simulink model "gridforMV"  (R2015b)
settings: Solver=FixedStepDiscrete  StartTime=0.0  StopTime=10.0  RelTol=1e-3
PreLoadFcn:
  | Ts=50e-6;
InitFcn:
  | Ts=50e-6;
undefined symbols (not defined in the file or in its folder): D1, Delta, DiscIntNeverNeededParam
libraries: powerlib x19, powerlib_meascontrol x5
Description:
  | Copyright 2008-2015 The MathWorks, Inc.
settings Model: FPTRunName=Active  Creator=MathWorks  LastModifiedBy=Eren
settings DataIOCC: SaveFormat=Array  SignalLoggingSaveFormat=ModelDataLogs
settings OptimizationCC: ExpressionDepthLimit=2147483647
settings DebuggingCC: UnderspecifiedInitializationDetection=Classic  MergeDetectMultiDrivingBlocksExec=none  SolverPrmCheckMsg=warning  FcnCallInpInsideContextMsg=EnableAllAsWarning  StateNameClashWarn=warning
settings HardwareCC: ProdBitPerPointer=32  ProdLargestAtomicFloat=None  ProdIntDivRoundTo=Undefined  ProdEndianess=Unspecified  ProdWordSize=32  ProdHWDeviceType=32-bit Generic
settings GRTTargetCC: GeneratePreprocessorConditionals=Disable all  CombineOutputUpdateFcns=off  GRTInterface=on
settings ConfigComp: CovModelRefEnable=Off  CovSFcnEnable=off

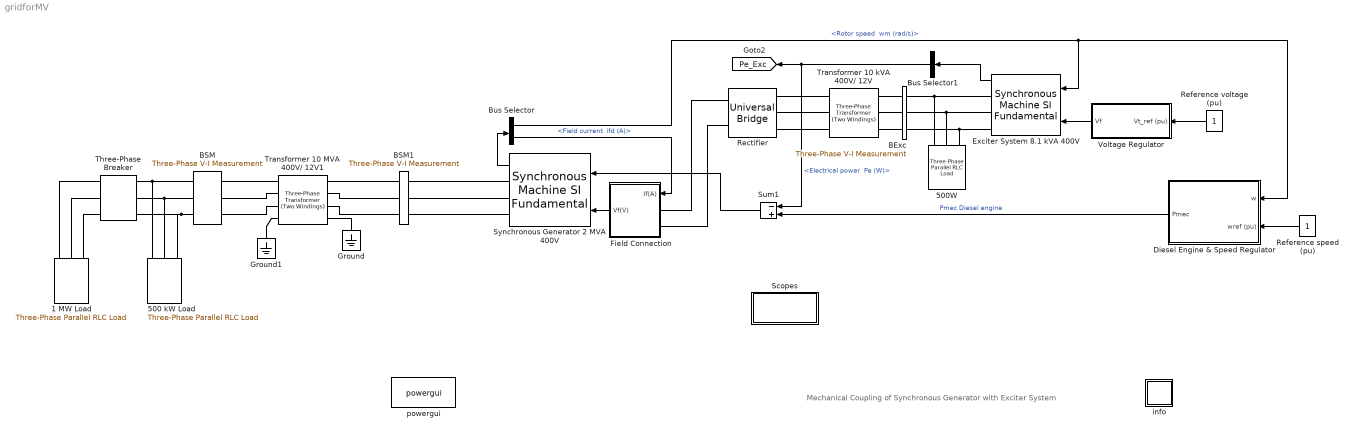
== system gridforMV ==
  note: Mechanical Coupling of Synchronous Generator with Exciter System
  "1 MW Load " : powerlib/Elements/Three-Phase Parallel RLC Load  LConnTagsString=A|B|C  Configuration=Y (grounded)  NominalVoltage=10800*sqrt(3)  Vabc=[1e3 1e3 1e3]  Vabcp=[1e3 1e3 1e3]  NominalFrequency=50  UnbalancedPower=off  ActivePower=1e6  InductivePower=0  CapacitivePower=0  Pabc=[10e3 9e3 11e3]  QLabc=[100 90 110]  QCabc=[100 90 110]  Pabcp=[10e3 9e3 11e3]  QLabcp=[100 90 110]  QCabcp=[100 90 110]  Measurements=None  LoadType=constant Z
  500 kW Load : powerlib/Elements/Three-Phase Parallel RLC Load  LConnTagsString=A|B|C  Configuration=Y (grounded)  NominalVoltage=10800*sqrt(3)  Vabc=[1e3 1e3 1e3]  Vabcp=[1e3 1e3 1e3]  NominalFrequency=50  UnbalancedPower=off  ActivePower=500e3  InductivePower=0  CapacitivePower=0  Pabc=[10e3 9e3 11e3]  QLabc=[100 90 110]  QCabc=[100 90 110]  Pabcp=[10e3 9e3 11e3]  QLabcp=[100 90 110]  QCabcp=[100 90 110]  Measurements=None  LoadType=constant Z
  500W : powerlib/Elements/Three-Phase Parallel RLC Load  LConnTagsString=A|B|C  Configuration=Y (grounded)  NominalVoltage=400  Vabc=[1e3 1e3 1e3]  Vabcp=[1e3 1e3 1e3]  NominalFrequency=50  UnbalancedPower=off  ActivePower=500  InductivePower=0  CapacitivePower=0  Pabc=[10e3 9e3 11e3]  QLabc=[100 90 110]  QCabc=[100 90 110]  Pabcp=[10e3 9e3 11e3]  QLabcp=[100 90 110]  QCabcp=[100 90 110]  Measurements=None  LoadType=constant Z
  BExc : powerlib/Measurements/Three-Phase V-I Measurement  VoltageMeasurement=phase-to-ground  SetLabelV=on  LabelV=Vabc_Exc  Vpu=on  VpuLL=off  CurrentMeasurement=yes  SetLabelI=on  LabelI=Iabc_Exc  Ipu=off  Pbase=100e6  Vbase=400  OutputType=Magnitude  PhasorSimulation=off  PSBequivalent=0
  BSM : powerlib/Measurements/Three-Phase V-I Measurement  VoltageMeasurement=phase-to-ground  SetLabelV=on  LabelV=Vabc_SMH  Vpu=off  VpuLL=off  CurrentMeasurement=yes  SetLabelI=on  LabelI=Iabc_SMH  Ipu=off  Pbase=1e3  Vbase=10800*sqrt(3)  OutputType=Magnitude  PhasorSimulation=off  PSBequivalent=0
  BSM1 : powerlib/Measurements/Three-Phase V-I Measurement  VoltageMeasurement=phase-to-ground  SetLabelV=on  LabelV=Vabc_SM  Vpu=off  VpuLL=off  CurrentMeasurement=yes  SetLabelI=on  LabelI=Iabc_SM  Ipu=off  Pbase=1e3  Vbase=10800*sqrt(3)  OutputType=Magnitude  PhasorSimulation=off  PSBequivalent=0
  Bus Selector : BusSelector  OutputSignals="Mechanical.Rotor speed  wm (rad/s),dq0 components.Field current  ifd (A)"
  Bus Selector1 : BusSelector  OutputSignals="Mechanical.Electrical power  Pe (W)"
  Diesel Engine & Speed Regulator : Subsystem  mask(Diesel Engine & Governor){Tr=[0.01 0.02 0.05], Ta=[0.25 0.009 0.0384], Tlim=[0.0  1.1], Td=0.024, Pm0=0.25, K=40, Ts=Ts}
      mask prompts: Tr "Regulator time constants [T1 T2 ] (s) :"; Ta "Actuator time constants [T3 T4 T5] (s) :"; Tlim "Torque limits [Tmin Tmax] (pu) :"; Td "Engine time delay Td (s) :"; Pm0 "Initial value of mechanical power  Pm0 (pu) :"; K "Regulator gain K:"; Ts "Sample time"
      mask help:
      | Diesel engine and governor system. The input 1 is the measured speed, in rad/s. The input 2 is the reference speed, in pu. The output is the mechanical power.
      |
      | Controller transfer function:
      | Hc=K.(1+T1.s)/(1+T2.s)
      |
      | Throttle actuator transfer function :
      | Ha= (1+T3.s) / [ (s (1+T4.s)(1+T5.s) ]
      |
      | Motor :
      | Time delay Td
      | Inertia and viscous friction are modeled in the Synchronous generator.
      |
      | The base power used to specify the initial mechanical power (Pm0 in pu) is the nominal power of the driven generator
  Exciter System 8.1 kVA 400V : powerlib/Machines/Synchronous Machine SI Fundamental  PresetModel=No  MechanicalLoad=Speed w  ShowDetailedParameters=on  RotorType=Salient-pole  Units=SI fundamental parameters  MeasurementBus=off  NominalParameters=[8100 400 50]  Stator=[1.62 0.004527 0.1086 0.05175]  Field=[1.208 0.01132]  Dampers2=[ 0.0664, 1.387e-3, 0.0292, 6.896e-4, 7.907e-3, 2.477e-3]  Dampers1=[3.142 0.007334 4.772 0.01015]  Mechanical=[0.2252 0.009 2]  PolePairs=2  InitialConditions=[0 -86.8318 1.02639 1.02639 1.02639 0.517558 -119.482 120.518 11.6647]  SetSaturation=off  Saturation=[695.64,774.7,917.5,1001.6,1082.2,1175.9,1293.6,1430.2,1583.7;9660,10623,12243,13063,13757,14437,15180,15890,16567]  DisplayVfd=off  LoadFlowParameters=[1,0,0,0,0]  TsPowergui=0  TsBlock=-1  IterativeModel=Trapezoidal non iterative  BusType=swing  Pref=0  Qref=0  Qmin=-inf  Qmax=inf  PLF=0  QLF=0
  Field Connection : Subsystem
  Ground : powerlib/Elements/Ground  LConnTagsString=a
  Ground1 : powerlib/Elements/Ground  LConnTagsString=a
  Rectifier : powerlib/Power Electronics/Universal Bridge  Arms=3  SnubberResistance=2  SnubberCapacitance=50e-6  Device=Diodes  Ron=1e-5  Lon=0  ForwardVoltages="[  0  0  ]"  ForwardVoltage=0  GTOparameters=[ 10e-6 , 20e-6 ]  IGBTparameters=[ 1e-6 , 2e-6 ]  Measurements=All voltages and currents  Measurements_2=None  converterType=Rectifier
  Reference speed (pu) : Constant
  Reference voltage (pu) : Constant
  Scopes : Subsystem
      mask Display: disp('Scopes')
  Sum1 : Sum  Inputs=-+
  Synchronous Generator 2 MVA 400V : powerlib/Machines/Synchronous Machine SI Fundamental  PresetModel=No  MechanicalLoad=Mechanical power Pm  ShowDetailedParameters=on  RotorType=Salient-pole  Units=SI fundamental parameters  MeasurementBus=off  NominalParameters="[2e+006 230 50  100]"  Stator=[0.00076 1.273e-005 0.0005246 0.0003845]  Field=[0.0001576 8.703e-005]  Dampers2=[ 0.0664, 1.387e-3, 0.0292, 6.896e-4, 7.907e-3, 2.477e-3]  Dampers1=[0.0161 0.0005447 0.002145 5.204e-005]  Mechanical="[56.29*2+.2252  0.8*2  2]"  PolePairs=2  InitialConditions=[0 -68.7412 1020.62 1020.62 1020.62 7.51406e-14 -120 120 10.4482]  SetSaturation=off  Saturation=[695.64,774.7,917.5,1001.6,1082.2,1175.9,1293.6,1430.2,1583.7;9660,10623,12243,13063,13757,14437,15180,15890,16567]  DisplayVfd=off  LoadFlowParameters=[1,0,0,0,0]  TsPowergui=0  TsBlock=-1  IterativeModel=Trapezoidal non iterative  BusType=swing  Pref=0  Qref=0  Qmin=-inf  Qmax=inf  PLF=0  QLF=0
  Three-Phase Breaker : powerlib/Elements/Three-Phase Breaker  InitialState=open  SwitchA=on  SwitchB=on  SwitchC=on  SwitchTimes=5  External=off  BreakerResistance=0.001  SnubberResistance=1e6  SnubberCapacitance=inf  Measurements=None
  Transformer 10 MVA 400V/ 12V1 : powerlib/Elements/Three-Phase Transformer (Two Windings)  Winding1Connection=Yn  Winding2Connection=Yn  CoreType=Three single-phase transformers  SetSaturation=off  Hysteresis=off  DataFile='hysteresis'  SetInitialFlux=off  Measurements=None  UNITS=pu  NominalPower=[ 13e6 , 50 ]  Winding1=[18706 0.001 0]  Winding2=[400 0.001 0]  Rm=Inf  Lm=Inf  L0=0.5  Saturation=[0 0;0.0023999 1.2;0.99999 1.52]  InitialFluxes=[0.80001 -0.80001 0.70001]  MoreParameters=off  BreakLoop=off  DataType=off  TransfoNumber=0
  Transformer 10 kVA 400V/ 12V : powerlib/Elements/Three-Phase Transformer (Two Windings)  Winding1Connection=Yg  Winding2Connection=Delta (D1)  CoreType=Three single-phase transformers  SetSaturation=off  Hysteresis=off  DataFile='hysteresis'  SetInitialFlux=off  Measurements=None  UNITS=pu  NominalPower=[ 10e3 , 50 ]  Winding1=[ 400 , 0.001 , 0 ]  Winding2=[ 12 , 0.001 , 0]  Rm=inf  Lm=inf  L0=0.5  Saturation=[ 0,0 ; 0.0024,1.2 ; 1.0,1.52 ]  InitialFluxes=[ 0.8 , -0.8 , 0.7 ]  MoreParameters=off  BreakLoop=off  DataType=off  TransfoNumber=0
  Voltage Regulator : Subsystem
      mask Display: disp('Voltage\nRegulator')
  info : Subsystem
      settings: OpenFcn=showdemo(bdroot(gcb))
      mask Display: disp('?')
  powergui : powerlib/powergui  SimulationMode=Discrete  SolverType=Tustin/Backward Euler (TBE)  SampleTime=Ts  frequency=60  SPID=off  DisableSnubberDevices=off  DisableRonSwitches=off  DisableVfSwitches=off  SwTol=0  DisplayEquations=off  Interpol=off  ExternalGateDelay=off  methode=off  Ts=0  FunctionMessages=off  echomessages=off  HookPort=off  EnableUseOfTLC=off  x0status=blocks  frequencyindice=50  Pbase=1e6  ErrMax=0.0001  Iterations=50  UnitsV=kV  UnitsW=kW  buscounter=0  RestoreLinks=warning  ResistiveCurrentMeasurement=off  Frange=[0:2:500]  Ylog=off  Xlog=on  ShowGrid=off  save=off  variable=ZData  structure=Ctrl_Sig  ZoomFFT=on  StartTime=0.0  cycles=1  DisplayStyle=1  fundamental=60  FreqAxis=off  MaxFrequency=1000  frequencyindicesteady=1  RmsSteady=1  display=off
  tag scope: Pe_Exc=global
  wires:
  Exciter System 8.1 kVA 400V/1 -> Bus Selector1/1
  Bus Selector1/1 -> [Pe_Exc], Sum1/1  "<Electrical power  Pe (W)>"
  Voltage Regulator/1(Vf) -> Exciter System 8.1 kVA 400V/2
  Field Connection/1(Vf(V)) -> Synchronous Generator 2 MVA 400V/2
  Reference voltage (pu)/1 -> Voltage Regulator/1(Vt_ref (pu))
  Reference speed (pu)/1 -> Diesel Engine & Speed Regulator/2(wref (pu))
  Sum1/1 -> Synchronous Generator 2 MVA 400V/1
  Diesel Engine & Speed Regulator/1(Pmec) -> Sum1/2  "Pmec Diesel engine"
  Synchronous Generator 2 MVA 400V/1 -> Bus Selector/1
  Bus Selector/2 -> Field Connection/1(If(A))  "<Field current  ifd (A)>"
  Bus Selector/1 -> Exciter System 8.1 kVA 400V/1, Diesel Engine & Speed Regulator/1(w)  "<Rotor speed  wm (rad/s)>"
  connections:
  Three-Phase Breaker/RConn1 -- 500 kW Load/LConn1 -- BSM/RConn1
  Three-Phase Breaker/RConn2 -- 500 kW Load/LConn2 -- BSM/RConn2
  BSM/RConn3 -- 500 kW Load/LConn3 -- Three-Phase Breaker/RConn3
  Transformer 10 kVA 400V/ 12V/RConn2 -- Rectifier/LConn2
  Transformer 10 kVA 400V/ 12V/RConn3 -- Rectifier/LConn3
  BExc/RConn1 -- Transformer 10 kVA 400V/ 12V/LConn1
  BExc/RConn2 -- Transformer 10 kVA 400V/ 12V/LConn2
  BExc/RConn3 -- Transformer 10 kVA 400V/ 12V/LConn3
  "1 MW Load "/LConn1 -- Three-Phase Breaker/LConn1
  "1 MW Load "/LConn2 -- Three-Phase Breaker/LConn2
  "1 MW Load "/LConn3 -- Three-Phase Breaker/LConn3
  Rectifier/RConn1 -- Field Connection/LConn1
  Rectifier/RConn2 -- Field Connection/LConn2
  Transformer 10 kVA 400V/ 12V/RConn1 -- Rectifier/LConn1
  BExc/LConn3 -- Exciter System 8.1 kVA 400V/RConn3 -- 500W/LConn3
  BExc/LConn2 -- Exciter System 8.1 kVA 400V/RConn2 -- 500W/LConn2
  BExc/LConn1 -- Exciter System 8.1 kVA 400V/RConn1 -- 500W/LConn1
  Transformer 10 MVA 400V/ 12V1/LConn2 -- BSM/LConn2
  Transformer 10 MVA 400V/ 12V1/LConn1 -- BSM/LConn1
  Transformer 10 MVA 400V/ 12V1/LConn3 -- BSM/LConn3
  BSM1/LConn1 -- Synchronous Generator 2 MVA 400V/RConn1
  BSM1/RConn1 -- Transformer 10 MVA 400V/ 12V1/RConn1
  BSM1/RConn2 -- Transformer 10 MVA 400V/ 12V1/RConn2
  BSM1/LConn2 -- Synchronous Generator 2 MVA 400V/RConn2
  BSM1/LConn3 -- Synchronous Generator 2 MVA 400V/RConn3
  BSM1/RConn3 -- Transformer 10 MVA 400V/ 12V1/RConn3
  Ground/LConn1 -- Transformer 10 MVA 400V/ 12V1/RConn4
  Ground1/LConn1 -- Transformer 10 MVA 400V/ 12V1/LConn4

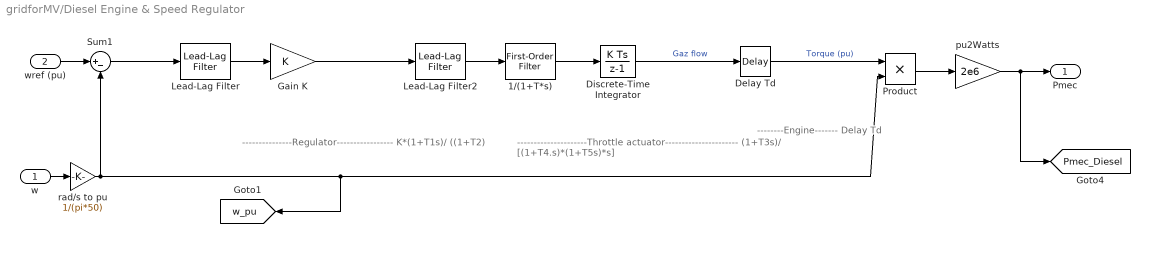
== system gridforMV/Diesel Engine & Speed Regulator ==
  note: ---------------------Throttle actuator----------------------
      | (1+T3s)/ [(1+T4.s)*(1+T5s)*s]
  note: ---------------Regulator-----------------
      | K*(1+T1s)/ ((1+T2)
  note: --------Engine-------
      | Delay Td
  w : Inport
  wref (pu) : Inport  Port=2
  1/(1+T*s) : powerlib_meascontrol/Filters/First-Order Filter  FilterType=Lowpass  Tc=Ta(3)  Ts=Ts  Initialize=on  Vac_Init=[0.8 -25 60]  Vdc_Init=-0.4  PlotResponse=off  FreqRange=[1 500 0.1]
  Delay Td : TransportDelay  DelayTime=Td  InitialOutput=Pm0
  Discrete-Time Integrator : DiscreteIntegrator  InitialCondition=Pm0  SampleTime=Ts  LimitOutput=on  UpperSaturationLimit=Tlim(2)  LowerSaturationLimit=Tlim(1)  ICPrevOutput=DiscIntNeverNeededParam  ICPrevScaledInput=DiscIntNeverNeededParam
  Gain K : Gain  Gain=K  SaturateOnIntegerOverflow=on  OutDataTypeStr=Inherit: Same as input  ParamDataTypeStr=Inherit: Same as input
  Lead-Lag Filter : powerlib_meascontrol/Filters/Lead-Lag Filter  T1=Tr(1)  T2=Tr(2)  Vdc_Init=0  Ts=Ts
  Lead-Lag Filter2 : powerlib_meascontrol/Filters/Lead-Lag Filter  T1=Ta(1)  T2=Ta(2)  Vdc_Init=0  Ts=Ts
  Product : Product  SaturateOnIntegerOverflow=on  InputSameDT=on  OutDataTypeStr=Inherit: Same as first input
  Sum1 : Sum  Inputs=|+-  SaturateOnIntegerOverflow=on
  pu2Watts : Gain  Gain=2e6
  rad/s to pu : Gain  Gain=1/(pi*50)
  Pmec : Outport  InitialOutput=0
  tag scope: Pmec_Diesel=global, w_pu=global
  wires:
  rad/s to pu/1 -> [w_pu], Product/2, Sum1/2
  pu2Watts/1 -> [Pmec_Diesel], Pmec/1
  Product/1 -> pu2Watts/1
  w/1 -> rad/s to pu/1
  Lead-Lag Filter/1 -> Gain K/1
  Delay Td/1 -> Product/1  "Torque (pu)"
  Discrete-Time Integrator/1 -> Delay Td/1  "Gaz flow"
  1/(1+T*s)/1 -> Discrete-Time Integrator/1
  Gain K/1 -> Lead-Lag Filter2/1
  Lead-Lag Filter2/1 -> 1/(1+T*s)/1
  Sum1/1 -> Lead-Lag Filter/1
  wref (pu)/1 -> Sum1/1

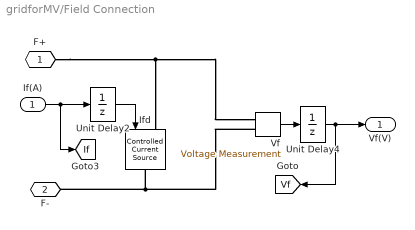
== system gridforMV/Field Connection ==
  If(A) : Inport
  Ifd : powerlib/Electrical Sources/Controlled Current Source  Initialize=on  Source_Type=DC  Amplitude=1.1254*100  Phase=0  Frequency=0  Measurements=None
  Unit Delay2 : UnitDelay  InitialCondition=1.1254*100  SampleTime=Ts
  Unit Delay4 : UnitDelay  InitialCondition=10.4482  SampleTime=Ts
  "Vf " : powerlib/Measurements/Voltage Measurement  PhasorSimulation=off  OutputType=Complex  PSBequivalent=0
  F+ : PMIOPort  Port=1  Side=Left
  F- : PMIOPort  Port=2  Side=Left
  Vf(V) : Outport
  tag scope: If=global, Vf=global
  wires:
  If(A)/1 -> Unit Delay2/1, [If]
  "Vf "/1 -> Unit Delay4/1
  Unit Delay2/1 -> Ifd/1
  Unit Delay4/1 -> Vf(V)/1, [Vf]
  connections:
  F+/RConn1 -- "Vf "/LConn1 -- Ifd/LConn1
  "Vf "/LConn2 -- Ifd/RConn1 -- F-/RConn1

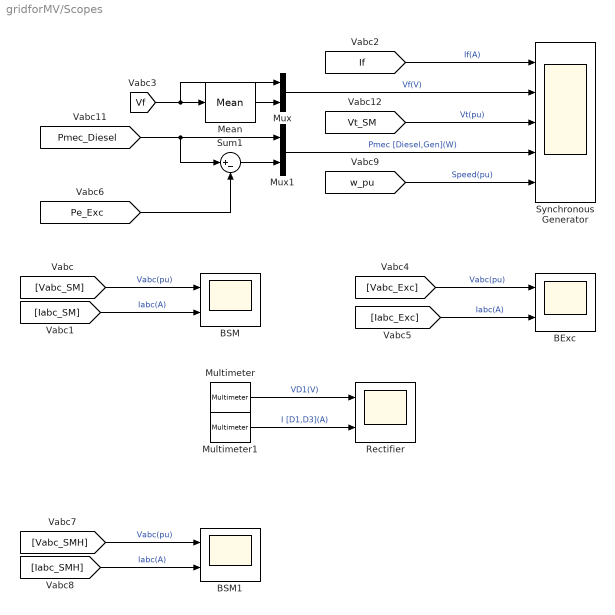
== system gridforMV/Scopes ==
  " BSM" : Scope  NumInputPorts=2
  " BSM1" : Scope  NumInputPorts=2
  " Rectifier" : Scope  NumInputPorts=2
  BExc : Scope  NumInputPorts=2
  Mean : powerlib_meascontrol/Measurements/Mean  Freq=50  Vinit=10.5  Ts=Ts
  Multimeter : powerlib/Measurements/Multimeter  PhasorSimulation=off  OutputType=Complex  sel=1  L=16  Gain=1  yselected={'Usw1: Rectifier'};  PSBOutputType=1  PSBequivalent=0  AxesSetting=[0,0.1,-100,100]  Display=0  SavedBlockNames=-11
  Multimeter1 : powerlib/Measurements/Multimeter  PhasorSimulation=off  OutputType=Complex  sel=[11 13]  L=16  Gain=[1 1]  yselected={'Isw1: Rectifier','Isw3: Rectifier'};  PSBOutputType=1  PSBequivalent=0  AxesSetting=[0,0.1,-100,100]  Display=0  SavedBlockNames=-11
  Mux : Mux  Inputs=2
  Mux1 : Mux  Inputs=2
  Sum1 : Sum  Inputs=|+-
  Synchronous Generator : Scope  NumInputPorts=5
  wires:
  [Vabc_SM] -> " BSM"/1  "Vabc(pu)"
  Multimeter/1 -> " Rectifier"/1  "VD1(V)"
  Multimeter1/1 -> " Rectifier"/2  "I [D1,D3](A)"
  [Vabc_Exc] -> BExc/1  "Vabc(pu)"
  [Iabc_Exc] -> BExc/2  "Iabc(A)"
  [Iabc_SM] -> " BSM"/2  "Iabc(A)"
  Mean/1 -> Mux/2
  Mux/1 -> Synchronous Generator/2  "Vf(V)"
  Mux1/1 -> Synchronous Generator/4  "Pmec [Diesel,Gen](W)"
  [w_pu] -> Synchronous Generator/5  "Speed(pu)"
  [Vt_SM] -> Synchronous Generator/3  "Vt(pu)"
  [If] -> Synchronous Generator/1  "If(A)"
  [Vf] -> Mean/1, Mux/1
  Sum1/1 -> Mux1/2
  [Pmec_Diesel] -> Mux1/1, Sum1/1
  [Pe_Exc] -> Sum1/2
  [Vabc_SMH] -> " BSM1"/1  "Vabc(pu)"
  [Iabc_SMH] -> " BSM1"/2  "Iabc(A)"

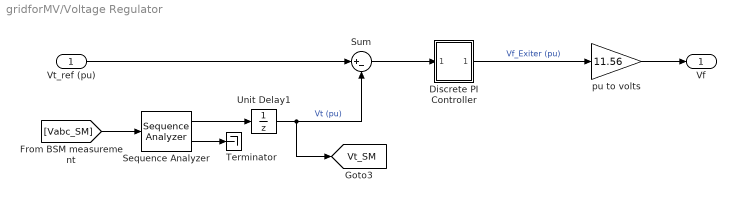
== system gridforMV/Voltage Regulator ==
  Vt_ref (pu) : Inport
  Discrete PI Controller : Subsystem  DialogController=POWERSYS.PowerSysDialog  mask(Discrete PI Controller){Kp=10, Ki=8, Par_Limits=[5  -5], Init=11.6647/11.56, Ts=Ts}
      mask prompts: Kp "Proportional gain (Kp):"; Ki "Integral gain (Ki):"; Par_Limits "Output limits: [ Upper   Lower ]"; Init "Output initial value:"; Ts "Sample time:"
      mask help: This block implements a discrete PI controller.
      mask init:
      | UpperLimit=Par_Limits(1);
      | LowerLimit=Par_Limits(2);
      | power_initmask();
      mask Display: disp('PI');
  Sequence Analyzer : powerlib_meascontrol/Measurements/Sequence Analyzer  Freq=50  n=1  seq=Positive  InInit=[1, 0]  Ts=50e-6
  Sum : Sum  Inputs=|+-
  Terminator : Terminator
  Unit Delay1 : UnitDelay  InitialCondition=1  SampleTime=Ts
  pu to volts : Gain  Gain=11.56
  Vf : Outport
  tag scope: Vt_SM=global
  wires:
  [Vabc_SM] -> Sequence Analyzer/1
  Sequence Analyzer/2 -> Terminator/1
  Sequence Analyzer/1 -> Unit Delay1/1
  Unit Delay1/1 -> [Vt_SM], Sum/2  "Vt (pu)"
  Sum/1 -> Discrete PI Controller/1(Error)
  Vt_ref (pu)/1 -> Sum/1
  Discrete PI Controller/1(Out) -> pu to volts/1  "Vf_Exiter (pu)"
  pu to volts/1 -> Vf/1

== system gridforMV/info ==

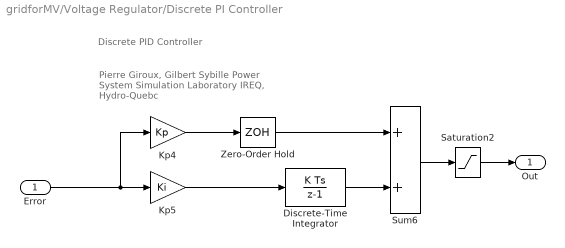
== system gridforMV/Voltage Regulator/Discrete PI Controller ==
  note: Discrete PID Controller
  note: Pierre Giroux, Gilbert Sybille
      | Power System Simulation Laboratory
      | IREQ, Hydro-Quebc
  Error : Inport  SampleTime=Ts
  Discrete-Time Integrator : DiscreteIntegrator  InitialCondition=Init  SampleTime=Ts  LimitOutput=on  UpperSaturationLimit=UpperLimit  LowerSaturationLimit=LowerLimit  ICPrevOutput=DiscIntNeverNeededParam  ICPrevScaledInput=DiscIntNeverNeededParam
  Kp4 : Gain  Gain=Kp  SampleTime=Ts  SaturateOnIntegerOverflow=on  OutDataTypeStr=Inherit: Same as input  ParamDataTypeStr=Inherit: Same as input
  Kp5 : Gain  Gain=Ki  SampleTime=Ts  SaturateOnIntegerOverflow=on  OutDataTypeStr=Inherit: Same as input  ParamDataTypeStr=Inherit: Same as input
  Saturation2 : Saturate  UpperLimit=UpperLimit  LowerLimit=LowerLimit  SampleTime=Ts
  Sum6 : Sum  SampleTime=Ts  SaturateOnIntegerOverflow=on  InputSameDT=on  OutDataTypeStr=Inherit: Same as first input
  Zero-Order Hold : ZeroOrderHold  SampleTime=Ts
  Out : Outport  SampleTime=Ts  InitialOutput=0
  wires:
  Zero-Order Hold/1 -> Sum6/1
  Saturation2/1 -> Out/1
  Discrete-Time Integrator/1 -> Sum6/2
  Kp4/1 -> Zero-Order Hold/1
  Kp5/1 -> Discrete-Time Integrator/1
  Sum6/1 -> Saturation2/1
  Error/1 -> Kp5/1, Kp4/1
